simulink model "vehicle_braking"  (R2021a)
settings: Solver=VariableStepAuto  StartTime=0  StopTime=80  RelTol=1e-3
values from neighbouring files (symbols this model uses):
  Ld = 0.3e-3    (= 0.0003)    [PMSM_paramaters.m]
  Lq = 0.4e-3    (= 0.0004)    [PMSM_paramaters.m]
  P = 4    [PMSM_paramaters.m]
  Pm = 0.15    [PMSM_paramaters.m]
  Rs = 0.03    [PMSM_paramaters.m]
  T_lookup = [289,289,0]    [PMSM_paramaters.m]
  Torque = 289    [PMSM_paramaters.m]
  Ts = 1e-2    (= 0.01)    [PMSM_paramaters.m]
undefined symbols (not defined in the file or in its folder): sigbuilder_block
libraries: spsSeriesRLCBranchLib x9, pid_lib x3, simulink x3, spsCurrentMeasurementLib x2, spsDCVoltageSourceLib x2, spsDiodeLib x2, spsMosfetLib x2, autolibshared x1, simulink_extras x1, spspowerguiLib x1
(part 2 of 2)

== system vehicle_braking/Vehicle Control Unit/Cruise Control/longitudinal driver/Subsystem ==
  v-nom : Inport
  e-ref : Inport  Port=2
  e-out : Inport  Port=3
  Divide2 : Product  Inputs=*/
  K-aw : Gain  Gain=0
  Ki : Gain
  Sum2 : Sum  Inputs=|++
  integral : Outport
  wires:
  Divide2/1 -> Sum2/1
  v-nom/1 -> Divide2/2
  e-ref/1 -> Ki/1
  K-aw/1 -> Sum2/2
  Ki/1 -> Divide2/1
  e-out/1 -> K-aw/1
  Sum2/1 -> integral/1
